simulink model "LKAS_AutoSave_20200909_1612"  (R2018b)
settings: Solver=FixedStepDiscrete  StartTime=0.0  StopTime=10.0  FixedStep=0.01  RelTol=1e-3
InitFcn:
  | tmpVer = ver('MATLAB');
  | tmpVer = str2num(tmpVer.Version);
  | % -------------------------------------------------------------------
  | %  MATLAB file generated by Simulink.saveVars on 21-Nov-2019 10:06:14
  | %  MATLAB version: 7.13.0.564 (R2011b)
  | % -------------------------------------------------------------------
  | 
  | 
  | SInt16 = Simulink.AliasType;
  | SInt16.Description = 'Num';
  | if (tmpVer > 7.11)
  | 	SInt16.DataScope = 'Auto';
  | end
  | SInt16.HeaderFile = 'Rte_Type.h';
  | SInt16.BaseType = 'int16';
  | 
  | SInt32 = Simulink.AliasType;
  | SInt32.Description = 'Num';
  | if (tmpVer > 7.11)
  | 	SInt32.DataScope = 'Auto';
  | end
  | SInt32.HeaderFile = 'Rte_Type.h';
  | SInt32.BaseType = 'int32';
  | 
  | SInt8 = Simulink.AliasType;
  | SInt8.Description = 'Num';
  | if (tmpVer > 7.11)
  | 	SInt8.DataScope = 'Auto';
  | end
  | SInt8.HeaderFile = 'Rte_Type.h';
  | SInt8.BaseType = 'int8';
  | 
  | T_A_m2_1024_1_u32 = Simulink.NumericType;
  | T_A_m2_1024_1_u32.Description = 'm2 (square meters  (m2))';
  | if (tmpVer > 7.11)
  | 	T_A_m2_1024_1_u32.DataScope = 'Auto';
  | end
  | T_A_m2_1024_1_u32.HeaderFile = 'Rte_Type.h';
  | T_A_m2_1024_1_u32.DataTypeMode = 'Fixed-point: slope and bias scaling';
  | T_A_m2_1024_1_u32.SignednessBool = false;
  | T_A_m2_1024_1_u32.WordLength = 32;
  | T_A_m2_1024_1_u32.FixedExponent = -10;
  | T_A_m2_1024_1_u32.SlopeAdjustmentFactor = 1;
  | T_A_m2_1024_1_u32.Bias = 0;
  | T_A_m2_1024_1_u32.DataTypeOverride = 'Inherit';
  | T_A_m2_1024_1_u32.IsAlias = true;
  | 
  | T_A_m2_65536_1_u16 = Simulink.NumericType;
  | T_A_m2_65536_1_u16.Description = 'm2 (square meters  (m2))';
  | if (tmpVer > 7.11)
  | 	T_A_m2_65536_1_u16.DataScope = 'Auto';
  | end
  | T_A_m2_65536_1_u16.HeaderFile = 'Rte_Type.h';
  | T_A_m2_65536_1_u16.DataTypeMode = 'Fixed-point: slope and bias scaling';
  | T_A_m2_65536_1_u16.SignednessBool = false;
  | T_A_m2_65536_1_u16.WordLength = 16;
  | T_A_m2_65536_1_u16.FixedExponent = -16;
  | T_A_m2_65536_1_u16.SlopeAdjustmentFactor = 1;
  | T_A_m2_65536_1_u16.Bias = 0;
  | T_A_m2_65536_1_u16.DataTypeOverride = 'Inherit';
  | ... (+4598 lines)
StopFcn:
  | clear  T_A_m2_1024_1_u32 T_A_m2_65536_1_u16 T_A_m2_Float32 T_A_mm2_10_1_u16 T_A_mm2_4_1_s16 T_A_mm2_Float32 T_Cnt_Num_10_1_u32 T_Cnt_Num_1_1_s16 T_Cnt_Num_1_1_s32 T_Cnt_Num_1_1_s8 T_Cnt_Num_1_1_u16 T_Cnt_Num_1_1_u32 T_Cnt_Num_1_1_u8 T_E_J_1_1_s32 T_E_J_Float32 T_E_kJ_128_1_s32 T_E_kJ_Float32 T_E_kwh_10_1_u16 T_E_kwh_Float32 T_Epl_kwhpkm_100_1_u16 T_Epl_kwhpkm_Float32 T_F_N_1_1_s16 T_F_N_Float32 T_I_A_1000_1_u16 T_I_A_1048576_1_s32 T_I_A_2048_1_s16 T_I_A_32_1_s16 T_I_A_Float32 T_I_mA_1_1_s16 T_I_mA_32768_128_s16 T_I_mA_Float32 T_J_kgpm2_128_1_u16 T_J_kgpm2_Float32 T_K_NA_1000_1_s16 T_K_NA_100_1_s16 T_K_NA_100_1_u16 T_K_NA_1024_1_s16 T_K_NA_1024_1_u16 T_K_NA_128_1_s16 T_K_NA_128_1_u16 T_K_NA_128_1_u8 T_K_NA_16777216_1_u32 T_K_NA_16_1_s16 T_K_NA_16_1_u16 T_K_NA_16_1_u8 T_K_NA_1_16_u16 T_K_NA_1_1_s16 T_K_NA_1_1_u16 T_K_NA_1_1_u8 T_K_NA_32768_1_s16 T_K_NA_32768_1_u16 T_K_NA_32_1_s8 T_K_NA_4096_1_u16 T_K_NA_4194304_1_s32 T_K_NA_4194304_1_u16 T_K_NA_65536_1_s32 T_K_NA_65536_1_u16 T_K_NA_8192_1_s16 T_K_NA_8_1_s16 T_K_NA_Float32 T_M_Nm_16_1_s16 T_M_Nm_1_1_s16 T_M_Nm_32768_1_s16 T_M_Nm_32_1_s16 T_M_Nm_4_1_s16 T_M_Nm_512_1_s16 T_M_Nm_Float32 T_P_W_1_4_s16 T_P_W_1_8_s16 T_P_W_Float32 T_P_kW_128_1_s16 T_P_kW_1_8_s16 T_P_kW_8_1_s32 T_P_kW_Float32 T_Pct_pct_1024_1_s32 T_Pct_pct_1024_1_u32 T_Pct_pct_10_1_s16 T_Pct_pct_10_1_u32 T_Pct_pct_128_100_s8 T_Pct_pct_1_1_s16 T_Pct_pct_1_4_u8 T_Pct_pct_255_100_u16 T_Pct_pct_255_100_u8 T_Pct_pct_256_1_s16 T_Pct_pct_256_1_u16 T_Pct_pct_65535_100_u16 T_Pct_pct_Float32 T_R_ohm_1024_1_s16 T_R_ohm_32_1_s16 T_R_ohm_Float32 T_TK_K_16_1_s16 T_TK_K_Float32 T_T_degC_10_400_1_u16 T_T_degC_16_1_s16 T_T_degC_1_40_1_u8 T_T_degC_2_80_1_u8 T_T_degC_Float32 T_U_V_1000_1_u16 T_U_V_10_1_u8 T_U_V_200_1_u8 T_U_V_32_1_s16 T_U_V_4096_1_s16 T_U_V_512_1_s16 T_U_V_65535_8_u16 T_U_V_8192_1_u16 T_U_V_Float32 T_U_mV_1_1_s16 T_U_mV_256_20_u16 T_U_mV_Float32 T_V_l_256_1_s16 T_V_l_4096_1_s16 T_V_l_64_1_s16 T_V_l_65535_100_u16 T_V_l_Float32 T_V_ml_128_1_s16 T_V_ml_1_1_s16 T_V_ml_32768_1_s16 T_V_ml_Float32 T_V_ul_32_1_u16 T_V_ul_Float32 T_Vpl_clpkm_512_1_u16 T_Vpl_clpkm_Float32 T_a_kphps_16_1_s16 T_a_kphps_Float32 T_a_mps2_128_1_s16 T_a_mps2_Float32 T_c_MJpkg_256_1_s16 T_c_MJpkg_Float32 T_c_kJpgpK_1024_1_s16 T_c_kJpgpK_Float32 T_c_kJpkgpK_128_1_u16 T_c_kJpkgpK_Float32 T_chrg_Ah_1_1_s16 T_chrg_Ah_1_1_u16 T_chrg_Ah_1_1_u8 T_chrg_Ah_256_1_u16 T_chrg_Ah_4194304_1_s32 T_chrg_Ah_512_1_u16 T_chrg_Ah_8_1_u16 T_chrg_Ah_Float32 T_cmp_NA_100_1_s16 T_cmp_NA_128_1_s16 T_cmp_NA_16_1_s16 T_cmp_NA_32768_1_u16 T_cmp_NA_Float32 T_d2n_rpmps2_4_1_s16 T_d2n_rpmps2_Float32 T_dPct_pctps_16_1_s16 T_dPct_pctps_256_1_s16 T_dPct_pctps_Float32 T_dT_degCps_128_1_s16 T_dT_degCps_Float32 T_dV_lph_1_1_s16 T_dV_lph_Float32 T_dV_lpm_128_1_s16 T_dV_lpm_32_1_s16 T_dV_lpm_Float32 T_dV_lps_1024_1_u16 T_dV_lps_4_1_u16 T_dV_lps_Float32 T_dV_mlps_1024_1_s16 T_dV_mlps_Float32 T_d_BitField16 T_dm_gps_128_1_s16 T_dm_gps_128_1_u16 T_dm_gps_256_1_u16 T_dm_gps_Float32 T_dm_mgps_1_1_s16 T_dm_mgps_Float32 T_dn_rpmps_1_1_s16 T_dn_rpmps_2_1_s16 T_dn_rpmps_Float32 T_dp_Paps_1_1_s16 T_dp_Paps_Float32 T_dp_kPaps_1_1_s16 T_dp_kPaps_8_1_s16 T_dp_kPaps_Float32 T_dphi_degps_128_1_s16 T_dphi_degps_8_1_s16 T_dphi_degps_Float32 T_dr_ps_256_1_s16 T_dr_ps_Float32 T_drho_mgplps_1_2_s16 T_drho_mgplps_Float32 T_e_NA_1_1_u8 T_f_Hz_1_1_u16 T_f_Hz_1_1_u32 T_f_Hz_64_1_u16 T_f_Hz_8_1_s16 T_f_Hz_Float32 T_g_BitField32 T_l_km_16_1_s16 T_l_km_1_1_u16 T_l_km_1_1_u32 T_l_km_Float32 T_l_m_1024_1_s16 T_l_m_16_1_s16 T_l_m_1_1_u32 T_l_m_Float32 T_l_mm_16_1_s16 T_l_mm_1_1_u16 T_l_mm_4096_1_s16 T_l_mm_4_1_u8 T_l_mm_64_1_s16 T_l_mm_Float32 T_m_g_1_1_s16 T_m_g_2048_1_s16 T_m_g_32_1_u16 T_m_g_Float32 T_m_kg_1024_1_s16 T_m_kg_1_1_s16 T_m_kg_1_1_u32 T_m_kg_Float32 T_m_mg_128_1_s16 T_m_mg_32_1_s16 T_m_mg_Float32 T_n_rpm_1_1_s16 T_n_rpm_1_25_u8 T_n_rpm_256_50_u16 T_n_rpm_2_25_u8 T_n_rpm_4_1_u16 T_n_rpm_Float32 T_p_MPa_64_1_s16 T_p_MPa_Float32 T_p_Pa_1_1_s16 T_p_Pa_Float32 T_p_kPa_1_10_u16 T_p_kPa_1_1_s16 T_p_kPa_1_1_u8 T_p_kPa_256_1_u16 T_p_kPa_32_1_u16 T_p_kPa_64_1_s16 T_p_kPa_Float32 T_phi_deg_100_1_s16 T_phi_deg_1024_1_s16 T_phi_deg_128_1_s16 T_phi_deg_1_1_u8 T_phi_deg_256_1_s16 T_phi_deg_2_1_s8 T_phi_deg_32_1_s16 T_phi_deg_512_6_s32 T_phi_deg_Float32 T_phi_rad_2048_1_s16 T_phi_rad_Float32 T_r_NA_1024_1_s16 T_r_NA_1024_1_u16 T_r_NA_16384_1_s16 T_r_NA_16_1_s16 T_r_NA_256_1_s8 T_r_NA_256_1_u16 T_r_NA_32768_1_u16 T_r_NA_32_1_u16 T_r_NA_4096_1_s16 T_r_NA_65535_2_u16 T_r_NA_8192_1_u16 T_r_NA_Float32 T_rho_gpl_8192_1_s16 T_rho_gpl_Float32 T_rho_kgpm3_16_1_s16 T_rho_kgpm3_Float32 T_rho_mgpl_1_1_s16 T_rho_mgpl_64_1_s16 T_rho_mgpl_Float32 T_t_hour_1_1_s16 T_t_hour_Float32 T_t_m_1_1_u16 T_t_m_Float32 T_t_ms_1_1_s16 T_t_ms_1_1_u16 T_t_ms_1_1_u32 T_t_ms_4096_1_s16 T_t_ms_64_1_s16 T_t_ms_Float32 T_t_s_1000_1_s16 T_t_s_100_1_s16 T_t_s_10_1_s16 T_t_s_10_1_u16 T_t_s_1_1_s16 T_t_s_1_1_u16 T_t_s_1_1_u32 T_t_s_Float32 T_t_us_10_1_u32 T_t_us_1_1_s16 T_t_us_1_1_u32 T_t_us_1_4_u16 T_t_us_Float32 T_v_kph_1_1_u8 T_v_kph_64_1_s16 T_v_kph_64_1_u16 T_v_kph_Float32 T_v_mps_256_1_s16 T_v_mps_Float32 T_w_radps_32_1_s16 T_w_radps_Float32 T_y_BitField8 T_y_BitFieldDiagProgress T_y_BitFieldDiagStatus T_y_NA_1_1_u8 SInt16 SInt32 SInt8 T_BOOLEAN UInt16 UInt32 UInt8 s16 s32 s8 u16 u32 u8
model workspace (MAT data in the model file):
  MCOS : class17 (value not decoded)
  MCOS : class17 (value not decoded)
  MCOS : class17 (value not decoded)
  MCOS : class17 (value not decoded)
  MCOS : class17 (value not decoded)
  MCOS : class17 (value not decoded)
  MCOS : class17 (value not decoded)
  MCOS : class17 (value not decoded)
  MCOS : class17 (value not decoded)
  MCOS : class17 (value not decoded)
  MCOS : class17 (value not decoded)
  MCOS : class17 (value not decoded)
  MCOS : class17 (value not decoded)
  MCOS : class17 (value not decoded)
  MCOS : class17 (value not decoded)
  MCOS : class17 (value not decoded)
  MCOS : class17 (value not decoded)
  MCOS : class17 (value not decoded)
  MCOS : class17 (value not decoded)
  MCOS : class17 (value not decoded)
  MCOS : class17 (value not decoded)
  MCOS : class17 (value not decoded)
  MCOS : class17 (value not decoded)
  MCOS : class17 (value not decoded)
  MCOS : class17 (value not decoded)
  MCOS : class17 (value not decoded)
  MCOS : class17 (value not decoded)
  MCOS : class17 (value not decoded)
  MCOS : class17 (value not decoded)
  MCOS : class17 (value not decoded)
  MCOS : class17 (value not decoded)
  MCOS : class17 (value not decoded)
  MCOS : class17 (value not decoded)
  MCOS : class17 (value not decoded)
  MCOS : class17 (value not decoded)
  MCOS : class17 (value not decoded)
  MCOS : class17 (value not decoded)
  MCOS : class17 (value not decoded)
  MCOS : class17 (value not decoded)
  MCOS : class17 (value not decoded)
  MCOS : class17 (value not decoded)
  MCOS : class17 (value not decoded)
  MCOS : class17 (value not decoded)
  MCOS : class17 (value not decoded)
  MCOS : class17 (value not decoded)
  MCOS : class17 (value not decoded)
  MCOS : class17 (value not decoded)
  MCOS : class17 (value not decoded)
  MCOS : class17 (value not decoded)
  MCOS : class17 (value not decoded)
  MCOS : class17 (value not decoded)
  MCOS : class17 (value not decoded)
  MCOS : class17 (value not decoded)
  MCOS : class17 (value not decoded)
  MCOS : class17 (value not decoded)
  MCOS : class17 (value not decoded)
  MCOS : class17 (value not decoded)
  MCOS : class17 (value not decoded)
  MCOS : class17 (value not decoded)
  MCOS : class17 (value not decoded)
  MCOS : class17 (value not decoded)
  MCOS : class17 (value not decoded)
  MCOS : class17 (value not decoded)
  MCOS : class17 (value not decoded)
  MCOS : class17 (value not decoded)
  MCOS : class17 (value not decoded)
  MCOS : class17 (value not decoded)
  MCOS : class17 (value not decoded)
  MCOS : class17 (value not decoded)
  MCOS : class17 (value not decoded)
  MCOS : class17 (value not decoded)
  MCOS : class17 (value not decoded)
  MCOS : class17 (value not decoded)
  MCOS : class17 (value not decoded)
  MCOS : class17 (value not decoded)
  MCOS : class17 (value not decoded)
  MCOS : class17 (value not decoded)
  MCOS : class17 (value not decoded)
  MCOS : class17 (value not decoded)
  MCOS : class17 (value not decoded)
  MCOS : class17 (value not decoded)
  MCOS : class17 (value not decoded)
  MCOS : class17 (value not decoded)
  MCOS : class17 (value not decoded)
  MCOS : class17 (value not decoded)
  MCOS : class17 (value not decoded)
  MCOS : class17 (value not decoded)
  MCOS : class17 (value not decoded)
  MCOS : class17 (value not decoded)
undefined symbols (not defined in the file): LKA_CarWidth, LKA_SampleTime, LKA_StrRatio_C, LKA_Veh2CamL_C, LKA_Veh2CamW_C, LKA_WhlBaseL_C, LL_CompSWA_C, LL_CrvtPrvwT_C, LL_DesDvt_C, LL_DvtComp_C, LL_DvtPrvwT_C, LL_DvtSpdDet_vDvtSpdMin_C, LL_HdAgExT_C, LL_HdAgPrvwT_C, LL_LAccMax_C, LL_LAccRMax_C, LL_LDW_EarliestWarnLine_C, LL_LDW_LatestWarnLine_C, LL_LDWS_SUPPRESS_HEADING, LL_LFClb_TFC_DiffCtlBalance, LL_LFClb_TFC_DiffCtrlMaxSWA, LL_LFClb_TFC_DiffCtrlRatio, LL_LFClb_TFC_facmGainLutGain1_C, LL_LFClb_TFC_facmGainLutGain2_C, LL_LFClb_TFC_facmIntegRatio, LL_LFClb_TFC_facmKlat_C, LL_LFClb_TFC_FfCtlRatio_C, LL_LFClb_TFC_phiIntegCtlMaxSWA_C, LL_LFClb_TFC_tiKlatPrvwT_C, LL_LFClb_TFC_vGainLutVehSpdLwr_C, LL_LFClb_TFC_vGainLutVehSpdUpr_C, LL_LKA_EarliestWarnLine_C, LL_LKA_LatestWarnLine_C, LL_LKAExPrcs_ExitC0Dvt, LL_LKAExPrcs_ExitC0Swt, LL_LKAExPrcs_tiExitTime1, LL_LKAExPrcs_tiExitTime2, LL_LKAExPrcs_tiExitTime3, LL_LKAS_OUT_OF_CONTROL_LAT_VEL, LL_LKAS_OUT_OF_CONTROL_TTLC, LL_LKASWASyn_M0, LL_LKASWASyn_M1, LL_LKASWASyn_M2, LL_LKASWASyn_M3K, LL_LKASWASyn_SWAaddMax, LL_LKASWASyn_T2, LL_LKASWASyn_tiTrqSwaRtTime, LL_LKASWASyn_tiTrqSwaTime, LL_LKASWASyn_TrqMax, LL_LKASWASyn_TrqSwaAddSwt, LL_LKASWASyn_TrqSwaRateDiff, LL_LSpdCompT_C, LL_lStpLngth_C, LL_MAX_DELAY_EPSSTAR_TIME, LL_MAX_DRIVER_TORQUE_DISABLE, LL_MAX_DRIVER_TORQUE_ENABLE, LL_MAX_LANE_WIDTH_DISABLE, LL_MAX_LANE_WIDTH_ENABLE, LL_MAX_LAT_ACC_DISABLE, LL_MAX_LAT_ACC_ENABLE ... (+29)
libraries: simulink x134, dspstat3 x3, simulink_extras x1
(part 8 of 19)

== system LKAS_AutoSave_20200909_1612/LKAS/LL/LL Inputs Mapping/bsLaneInfo/LanesReconstruct /Left 1Lane Reconstruct (Lft1LaneR) ==
  stFlag : Inport
  bsL1Info : Inport  Port=2
  Bus Creator2 : BusCreator  Inputs=10
  Bus Selector1 : BusSelector  OutputSignals=L1_C0,L1_C1,L1_C2,L1_C3,L1_VR,L1_Q,L1_Type,L1_W,L1_TLC,L1_LC
  Constant : Constant  Value=0  OutDataTypeStr=uint16
  Switch3 : Switch  Criteria=u2 > Threshold
  bsL1InfoR : Outport
  wires:
  Bus Selector1/9 -> Bus Creator2/9  "<L1_TLC>"
  Bus Selector1/10 -> Bus Creator2/10  "<L1_LC>"
  Bus Selector1/8 -> Bus Creator2/8  "<L1_W>"
  Bus Selector1/7 -> Bus Creator2/7  "<L1_Type>"
  Bus Selector1/5 -> Bus Creator2/5  "<L1_VR>"
  bsL1Info/1 -> Bus Selector1/1
  stFlag/1 -> Switch3/2
  Bus Selector1/6 -> Switch3/1  "<L1_Q>"
  Constant/1 -> Switch3/3
  Switch3/1 -> Bus Creator2/6  "L1_Q"
  Bus Creator2/1 -> bsL1InfoR/1  "bsL1Info"
  Bus Selector1/4 -> Bus Creator2/4  "<L1_C3>"
  Bus Selector1/3 -> Bus Creator2/3  "<L1_C2>"
  Bus Selector1/2 -> Bus Creator2/2  "<L1_C1>"
  Bus Selector1/1 -> Bus Creator2/1  "<L1_C0>"

== system LKAS_AutoSave_20200909_1612/LKAS/LL/LL Inputs Mapping/bsLaneInfo/LanesReconstruct /Left Lane Reconstruct (LftLaneR) ==
  lRoadW : Inport
  bsR0Info : Inport  Port=2
  bsL0Info : Inport  Port=3
  Add : Sum  Inputs=+-  OutDataTypeStr=single
  Bus Creator : BusCreator  Inputs=10
  Bus Selector1 : BusSelector  OutputSignals=L0_Q
  Bus Selector3 : BusSelector  OutputSignals=R0_C0,R0_C1,R0_C2,R0_C3,R0_VR,R0_Type,R0_W,R0_TLC,R0_LC
  Cast To Single{1..4,6..7} (6 alike) : DataTypeConversion  OutDataTypeStr=single  LockScale=on
  Cast To Single5 : DataTypeConversion  OutDataTypeStr=uint8  LockScale=on
  Cast To Single8 : DataTypeConversion  OutDataTypeStr=uint8  LockScale=on
  Gain : Gain  Gain=-1  OutDataTypeStr=Inherit: Same as input
  bsL0InfoR : Outport
  wires:
  Cast To Single7/1 -> Bus Creator/9  "L0_TLC"
  Cast To Single8/1 -> Bus Creator/10  "L0_LC"
  Cast To Single4/1 -> Bus Creator/5  "L0_VR"
  Cast To Single6/1 -> Bus Creator/8  "L0_W"
  Cast To Single5/1 -> Bus Creator/7  "L0_Type"
  Bus Selector3/8 -> Cast To Single7/1  "<R0_TLC>"
  Bus Selector3/9 -> Cast To Single8/1  "<R0_LC>"
  Bus Selector3/7 -> Cast To Single6/1  "<R0_W>"
  Bus Selector3/6 -> Cast To Single5/1  "<R0_Type>"
  lRoadW/1 -> Add/1
  bsR0Info/1 -> Bus Selector3/1
  Bus Selector3/1 -> Add/2  "<R0_C0>"
  Add/1 -> Gain/1
  Bus Selector3/2 -> Cast To Single1/1  "<R0_C1>"
  Bus Selector3/3 -> Cast To Single2/1  "<R0_C2>"
  Bus Selector3/4 -> Cast To Single3/1  "<R0_C3>"
  Bus Selector3/5 -> Cast To Single4/1  "<R0_VR>"
  bsL0Info/1 -> Bus Selector1/1
  Bus Selector1/1 -> Bus Creator/6  "<L0_Q>"
  Gain/1 -> Bus Creator/1  "L0_C0"
  Cast To Single1/1 -> Bus Creator/2  "L0_C1"
  Cast To Single2/1 -> Bus Creator/3  "L0_C2"
  Cast To Single3/1 -> Bus Creator/4  "L0_C3"
  Bus Creator/1 -> bsL0InfoR/1  "bsL0Info"

== system LKAS_AutoSave_20200909_1612/LKAS/LL/LL Inputs Mapping/bsLaneInfo/LanesReconstruct /Right 1Lane Reconstruct (Rgt1LaneR) ==
  stFlag : Inport
  bsR1Info : Inport  Port=2
  Bus Creator3 : BusCreator  Inputs=10
  Bus Selector1 : BusSelector  OutputSignals=R1_C0,R1_C1,R1_C2,R1_C3,R1_VR,R1_Q,R1_Type,R1_W,R1_TLC,R1_LC
  Constant : Constant  Value=0  OutDataTypeStr=uint16
  Switch3 : Switch  Criteria=u2 > Threshold
  bsL1InfoR : Outport
  wires:
  Bus Selector1/9 -> Bus Creator3/9  "<R1_TLC>"
  Bus Selector1/10 -> Bus Creator3/10  "<R1_LC>"
  Bus Selector1/8 -> Bus Creator3/8  "<R1_W>"
  Bus Selector1/7 -> Bus Creator3/7  "<R1_Type>"
  Bus Selector1/5 -> Bus Creator3/5  "<R1_VR>"
  Bus Selector1/1 -> Bus Creator3/1  "<R1_C0>"
  Bus Selector1/2 -> Bus Creator3/2  "<R1_C1>"
  Bus Selector1/3 -> Bus Creator3/3  "<R1_C2>"
  Bus Selector1/4 -> Bus Creator3/4  "<R1_C3>"
  Constant/1 -> Switch3/3
  Bus Selector1/6 -> Switch3/1  "<R1_Q>"
  stFlag/1 -> Switch3/2
  bsR1Info/1 -> Bus Selector1/1
  Bus Creator3/1 -> bsL1InfoR/1  "bsR1Info"
  Switch3/1 -> Bus Creator3/6  "R1_Q"

== system LKAS_AutoSave_20200909_1612/LKAS/LL/LL Inputs Mapping/bsLaneInfo/LanesReconstruct /Right Lane Reconstruct (RgtLaneR) ==
  bsL0Info : Inport
  bsR0Info : Inport  Port=2
  lRoadW : Inport  Port=3
  Add : Sum  OutDataTypeStr=single
  Bus Creator1 : BusCreator  Inputs=10
  Bus Selector1 : BusSelector  OutputSignals=R0_Q
  Bus Selector3 : BusSelector  OutputSignals=L0_C0,L0_C1,L0_C2,L0_C3,L0_VR,L0_Type,L0_W,L0_TLC,L0_LC
  Cast To Single{1..4,6..7} (6 alike) : DataTypeConversion  OutDataTypeStr=single  LockScale=on
  Cast To Single5 : DataTypeConversion  OutDataTypeStr=uint8  LockScale=on
  Cast To Single8 : DataTypeConversion  OutDataTypeStr=uint8  LockScale=on
  bsR0InfoR : Outport
  wires:
  Cast To Single7/1 -> Bus Creator1/9  "R0_TLC"
  Cast To Single6/1 -> Bus Creator1/8  "R0_W"
  Cast To Single8/1 -> Bus Creator1/10  "R0_LC"
  Cast To Single5/1 -> Bus Creator1/7  "R0_Type"
  Bus Selector3/8 -> Cast To Single7/1  "<L0_TLC>"
  Bus Selector3/9 -> Cast To Single8/1  "<L0_LC>"
  Bus Selector3/7 -> Cast To Single6/1  "<L0_W>"
  Bus Selector3/6 -> Cast To Single5/1  "<L0_Type>"
  Bus Selector3/1 -> Add/2  "<L0_C0>"
  bsL0Info/1 -> Bus Selector3/1
  lRoadW/1 -> Add/1
  Bus Selector3/2 -> Cast To Single1/1  "<L0_C1>"
  Bus Selector3/3 -> Cast To Single2/1  "<L0_C2>"
  Bus Selector3/4 -> Cast To Single3/1  "<L0_C3>"
  Bus Selector3/5 -> Cast To Single4/1  "<L0_VR>"
  bsR0Info/1 -> Bus Selector1/1
  Bus Selector1/1 -> Bus Creator1/6  "<R0_Q>"
  Bus Creator1/1 -> bsR0InfoR/1  "bsR0Info"
  Add/1 -> Bus Creator1/1  "R0_C0"
  Cast To Single1/1 -> Bus Creator1/2  "R0_C1"
  Cast To Single2/1 -> Bus Creator1/3  "R0_C2"
  Cast To Single3/1 -> Bus Creator1/4  "R0_C3"
  Cast To Single4/1 -> Bus Creator1/5  "R0_VR"

== system LKAS_AutoSave_20200909_1612/LKAS/LL/LL Inputs Mapping/bsLaneInfo/LanesReconstruct /RoadSide Offset ==
  bsL0Info : Inport
  bsR0Info : Inport  Port=2
  Abs : Abs
  Add : Sum
  Add1 : Sum  Inputs=+-
  Add2 : Sum
  Average Filter (AvrgFlt) : Subsystem
      mask Display:
      | port_label('input', 1, 'In');
      | port_label('input', 2, 'PtsNum');
      | port_label('output', 1, 'Out');
      | color('blue');
      | text(0.98,0.9,'VCDC Block','horizontalAlignment','right');
      | color('black');
      | text(0.5,0.55,'Average Filter','horizontalAlignment','center');
      | text(0.5,0.4,'(AvrgFlt)','horizontalAlignment','center');
  Average Filter (AvrgFlt)1 : Subsystem
      mask Display:
      | port_label('input', 1, 'In');
      | port_label('input', 2, 'PtsNum');
      | port_label('output', 1, 'Out');
      | color('blue');
      | text(0.98,0.9,'VCDC Block','horizontalAlignment','right');
      | color('black');
      | text(0.5,0.55,'Average Filter','horizontalAlignment','center');
      | text(0.5,0.4,'(AvrgFlt)','horizontalAlignment','center');
  Bus Creator1 : BusCreator  Inputs=10
  Bus Creator2 : BusCreator  Inputs=10
  Bus Selector1 : BusSelector  OutputSignals=R0_C0,R0_C1,R0_C2,R0_C3,R0_VR,R0_Q,R0_Type,R0_W,R0_TLC,R0_LC
  Bus Selector3 : BusSelector  OutputSignals=L0_C0,L0_C1,L0_C2,L0_C3,L0_VR,L0_Q,L0_Type,L0_W,L0_TLC,L0_LC
  Compare To Constant : simulink/Logic and Bit Operations/Compare To Constant  relop===  const=2  OutDataTypeStr=boolean
  Compare To Constant1 : simulink/Logic and Bit Operations/Compare To Constant  relop===  const=2  OutDataTypeStr=boolean
  PtsNum : Constant  Value=10  OutDataTypeStr=single
  PtsNum1 : Constant  Value=10  OutDataTypeStr=single
  Road Width Calculation (RoadWCal) : Subsystem
  Saturation : Saturate  UpperLimit=0.004  LowerLimit=0
  Switch : Switch  Criteria=u2 > Threshold
  Switch1 : Switch  Criteria=u2 > Threshold
  get_roadside_offset : MATLAB Function  TreatAsAtomicUnit=on
  bsL0Infoout : Outport
  bsR0Infoout : Outport  Port=2
  lRoadW : Outport  Port=3
  wires:
  Bus Selector3/9 -> Bus Creator1/9  "<L0_TLC>"
  Bus Creator1/1 -> bsL0Infoout/1  "bsL0Info"
  bsL0Info/1 -> Road Width Calculation (RoadWCal)/1(RoadWCal_L0Info), Bus Selector3/1
  Bus Selector3/1 -> Switch/3, Add/1  "<L0_C0>"
  Bus Selector3/2 -> Bus Creator1/2  "<L0_C1>"
  Bus Selector3/3 -> Bus Creator1/3, Add2/1  "<L0_C2>"
  Bus Selector3/4 -> Bus Creator1/4  "<L0_C3>"
  Bus Selector3/6 -> Bus Creator1/6  "<L0_Q>"
  Bus Selector3/5 -> Bus Creator1/5  "<L0_VR>"
  Bus Selector3/7 -> Bus Creator1/7, Compare To Constant/1  "<L0_Type>"
  Bus Selector3/8 -> Bus Creator1/8  "<L0_W>"
  Bus Selector3/10 -> Bus Creator1/10  "<L0_LC>"
  Compare To Constant/1 -> Switch/2
  [offset] -> Add/2
  Add/1 -> Switch/1
  Average Filter (AvrgFlt)/1(Out) -> Bus Creator1/1  "L0_C0"
  Bus Selector1/9 -> Bus Creator2/9  "<R0_TLC>"
  Bus Selector1/3 -> Bus Creator2/3, Add2/2  "<R0_C2>"
  bsR0Info/1 -> Road Width Calculation (RoadWCal)/2(RoadWCal_R0Info), Bus Selector1/1
  Bus Selector1/5 -> Bus Creator2/5  "<R0_VR>"
  Bus Selector1/2 -> Bus Creator2/2  "<R0_C1>"
  Bus Creator2/1 -> bsR0Infoout/1  "bsR0Info"
  Bus Selector1/4 -> Bus Creator2/4  "<R0_C3>"
  Bus Selector1/6 -> Bus Creator2/6  "<R0_Q>"
  Bus Selector1/10 -> Bus Creator2/10  "<R0_LC>"
  Bus Selector1/7 -> Bus Creator2/7, Compare To Constant1/1  "<R0_Type>"
  Add1/1 -> Switch1/1
  Bus Selector1/8 -> Bus Creator2/8  "<R0_W>"
  Average Filter (AvrgFlt)1/1(Out) -> Bus Creator2/1  "R0_C0"
  Compare To Constant1/1 -> Switch1/2
  [offset] -> Add1/2
  Bus Selector1/1 -> Switch1/3, Add1/1  "<R0_C0>"
  Road Width Calculation (RoadWCal)/1(RoadWCal_lRoadW) -> lRoadW/1, get_roadside_offset/2(lanewidth)
  Add2/1 -> Abs/1
  Abs/1 -> Saturation/1
  Saturation/1 -> get_roadside_offset/1(cur)
  get_roadside_offset/1(offset) -> [offset]
  Switch/1 -> Average Filter (AvrgFlt)/1(In)
  PtsNum/1 -> Average Filter (AvrgFlt)/2(PtsNum)
  Switch1/1 -> Average Filter (AvrgFlt)1/1(In)
  PtsNum1/1 -> Average Filter (AvrgFlt)1/2(PtsNum)

== system LKAS_AutoSave_20200909_1612/LKAS/LL/LLOn/LDW/Heading Angle Detection (HdAgDet)/If Action Subsystem ==
  In1 : Inport
  Action Port : ActionPort  InitializeStates=reset  ActionType=then
  Gain : Gain  Gain=-1  OutDataTypeStr=single
  rad to deg : Gain  Gain=180/pi  OutDataTypeStr=single
  Out1 : Outport  InitialOutput=0
  wires:
  In1/1 -> Gain/1
  Gain/1 -> rad to deg/1
  rad to deg/1 -> Out1/1

== system LKAS_AutoSave_20200909_1612/LKAS/LL/LLOn/LDW/Heading Angle Detection (HdAgDet)/If Action Subsystem1 ==
  In1 : Inport
  Action Port : ActionPort  InitializeStates=reset  ActionType=elseif
  rad to deg : Gain  Gain=180/pi  OutDataTypeStr=single
  Out1 : Outport  InitialOutput=0
  wires:
  In1/1 -> rad to deg/1
  rad to deg/1 -> Out1/1

== system LKAS_AutoSave_20200909_1612/LKAS/LL/LLOn/LDW/Heading Angle Detection (HdAgDet)/If Action Subsystem2 ==
  Action Port : ActionPort  InitializeStates=reset  ActionType=else
  Constant : Constant  Value=0  OutDataTypeStr=single
  Out1 : Outport  InitialOutput=0
  wires:
  Constant/1 -> Out1/1

== system LKAS_AutoSave_20200909_1612/LKAS/LL/LLOn/LDW/Heading Angle Detection (HdAgDet)/Sum Condition ==
  In : Inport
  Sum : Inport  Port=2
  state = reset : EnablePort  StatesWhenEnabling=reset
  Add1 : Sum  OutDataTypeStr=single
  Data Type Conversion : DataTypeConversion  OutDataTypeStr=uint8
  Memory : Memory  InheritSampleTime=on
  Relational Operator : RelationalOperator  OutDataTypeStr=boolean  RndMeth=Nearest
  Saturation : Saturate  UpperLimit=600  LowerLimit=0
  Out : Outport  OutputWhenDisabled=reset  InitialOutput=0
  wires:
  Relational Operator/1 -> Data Type Conversion/1
  Memory/1 -> Add1/2
  Add1/1 -> Saturation/1
  In/1 -> Add1/1
  Sum/1 -> Relational Operator/2
  Data Type Conversion/1 -> Out/1
  Saturation/1 -> Memory/1, Relational Operator/1

== system LKAS_AutoSave_20200909_1612/LKAS/LL/LLOn/LKA/Driver Torque Addition (DTA)/Subsystem ==
  DTA_bsInInfoSyn : Inport
  DTA_bsLFClb : Inport  Port=2
  LKA_SampleTime : Inport  Port=3
  Enable : EnablePort
  Add : Sum
  Bus Selector2 : BusSelector  OutputSignals=bsVehMovInfo.ESC_VehSpd,bsEPSInfo.EPS_SW_Trq,bsLaneInfo.bsL0Info.L0_C0,bsLaneInfo.bsR0Info.R0_C0
  Bus Selector4 : BusSelector  OutputSignals=LL_LKASWAClb.LL_LKASWASyn_SWAaddMax,LL_LKASWAClb.LL_LKASWASyn_TrqMax,LL_LKASWAClb.LL_LKASWASyn_TrqSwaAddSwt,LL_LKASWAClb.LL_LKASWASyn_tiTrqSwaTime,LL_LKASWAClb.LL_LKASWASyn_tiTrqSwaRtTime,LL_LKASWAClb.LL_LKASWASyn_TrqSwaRateDiff
  Constant1 : Constant  Value=5  OutDataTypeStr=single
  Constant2 : Constant  Value=-5  OutDataTypeStr=single
  Divide1 : Product  Inputs=***
  Divide3 : Product  Inputs=**
  DriverSwaTrqAdd : MATLAB Function  TreatAsAtomicUnit=on
  LowPass : Subsystem
  LowPass1 : Subsystem
  Rate Limiter Dynamic : simulink/Discontinuities/Rate Limiter Dynamic
      settings: SourceProductName=Simulink
  Saturation : Saturate  UpperLimit=30  LowerLimit=-30
  Out1 : Outport  OutputWhenDisabled=reset  InitialOutput=0
  wires:
  Add/1 -> Rate Limiter Dynamic/2
  Bus Selector4/3 -> Divide3/1, Divide1/1  "<LL_LKASWASyn_TrqSwaAddSwt>"
  LowPass1/1(y) -> Saturation/1  "SWARateAdd"
  Divide3/1 -> Add/1  "TrqSWAAdd"
  Constant2/1 -> Rate Limiter Dynamic/3
  Bus Selector4/1 -> DriverSwaTrqAdd/5(swaaddmax)  "<LL_LKASWASyn_SWAaddMax>"
  Constant1/1 -> Rate Limiter Dynamic/1
  DriverSwaTrqAdd/1(Swaadd) -> LowPass/2(u)  "TrqSWAAddRaw"
  Rate Limiter Dynamic/1 -> Out1/1
  Saturation/1 -> Divide1/2
  DTA_bsInInfoSyn/1 -> Bus Selector2/1
  Bus Selector4/4 -> LowPass/1(T)  "<LL_LKASWASyn_tiTrqSwaTime>"
  LowPass/1(y) -> Divide3/2, LowPass1/2(u)  "TrqSWAAdd"
  Divide1/1 -> Add/2  "SWARateAdd"
  Bus Selector2/2 -> DriverSwaTrqAdd/2(trq)  "<EPS_SW_Trq>"
  Bus Selector2/4 -> DriverSwaTrqAdd/4(r0c0)  "<R0_C0>"
  Bus Selector4/6 -> Divide1/3  "<LL_LKASWASyn_TrqSwaRateDiff>"
  Bus Selector2/1 -> DriverSwaTrqAdd/1(spd)  "<ESC_VehSpd>"
  Bus Selector4/5 -> LowPass1/1(T)  "<LL_LKASWASyn_tiTrqSwaRtTime>"
  Bus Selector2/3 -> DriverSwaTrqAdd/3(l0c0)  "<L0_C0>"
  LKA_SampleTime/1 -> LowPass/3(dT), LowPass1/3(dT)
  Bus Selector4/2 -> DriverSwaTrqAdd/6(trqmax)  "<LL_LKASWASyn_TrqMax>"
  DTA_bsLFClb/1 -> Bus Selector4/1

== system LKAS_AutoSave_20200909_1612/LKAS/LL/LLOn/LKA/Driver Torque Addition (DTA)/Subsystem1 ==
  DTA_bsInInfoSyn : Inport
  DTA_bsLFClb : Inport  Port=2
  Add1 : Sum  Inputs=-+
  Bus Selector : BusSelector  OutputSignals=bsEPSInfo.EPS_SW_Trq
  Bus Selector1 : BusSelector  OutputSignals=LL_LKASWAClb.LL_LKASWASyn_M3K,LL_LKASWAClb.LL_LKASWASyn_M0,LL_LKASWAClb.LL_LKASWASyn_M1,LL_LKASWAClb.LL_LKASWASyn_M2,LL_LKASWAClb.LL_LKASWASyn_T2
  Divide : Product  Inputs=**
  MATLAB Function : MATLAB Function  TreatAsAtomicUnit=on
  Moving Standard Deviation2 : Subsystem  TreatAsAtomicUnit=on
      mask Display: disp(['Moving' char(10) 'Standard' char(10) 'Deviation']);
  Saturation1 : Saturate  UpperLimit=0.2  LowerLimit=0
  Saturation2 : Saturate  UpperLimit=1  LowerLimit=0
  TickTime (TTime) : Subsystem
      mask Display:
      | port_label('output', 1, 'TTime');
      | color('blue');
      | text(0.98,0.9,'VCDC Block','horizontalAlignment','right');
      | color('black');
      | text(0.5,0.55,'Tick Time','horizontalAlignment','center');
      | text(0.5,0.4,'(TTime)','horizontalAlignment','center');
  Out1 : Outport
  wires:
  Bus Selector1/2 -> MATLAB Function/1(M0)  "<LL_LKASWASyn_M0>"
  Bus Selector1/3 -> MATLAB Function/2(M1)  "<LL_LKASWASyn_M1>"
  [PT1] -> MATLAB Function/4(T1)
  [T] -> MATLAB Function/6(T)
  Saturation1/1 -> Add1/1  "M3"
  MATLAB Function/1(M) -> Add1/2
  Bus Selector1/5 -> MATLAB Function/5(T2)  "<LL_LKASWASyn_T2>"
  TickTime (TTime)/1(Out1) -> [T]
  Divide/1 -> Saturation1/1
  Add1/1 -> Saturation2/1
  Bus Selector1/1 -> Divide/2  "<LL_LKASWASyn_M3K>"
  Bus Selector1/4 -> MATLAB Function/3(M2)  "<LL_LKASWASyn_M2>"
  Bus Selector/1 -> Moving Standard Deviation2/1(In1)  "<EPS_SW_Trq>"
  Moving Standard Deviation2/1(Out1) -> Divide/1
  DTA_bsInInfoSyn/1 -> Bus Selector/1
  DTA_bsLFClb/1 -> Bus Selector1/1
  Saturation2/1 -> Out1/1

== system LKAS_AutoSave_20200909_1612/LKAS/LL/LLOn/LKA/LKA Exit Processing (LKAExPrcs)/Exit Time 1 ==
  bsLKAInPInfo : Inport
  bsLKAClb : Inport  Port=2
  Abs : Abs
  Add : Sum
  Add2 : Sum  OutDataTypeStr=single
  Bus Selector1 : BusSelector  OutputSignals=LL_LKAExPrcs.LL_LKAExPrcs_tiExitTime1
  Bus Selector2 : BusSelector  OutputSignals=Pr_bsPrInfo.bsPrCrvtInfo.crPrvwCrvt
  Constant : Constant  Value=0.004  OutDataTypeStr=single
  Constant1 : Constant  Value=0.5  OutDataTypeStr=single
  Divide : Product  Inputs=***/
  Memory : Memory  InheritSampleTime=on
  Relational Operator4 : RelationalOperator  OutDataTypeStr=boolean  RndMeth=Nearest
  Saturation : Saturate  UpperLimit=0.004  LowerLimit=0
  Saturation2 : Saturate  UpperLimit=10  LowerLimit=0
  Exit1 : Outport
  wires:
  [LKA_SampleTime] -> Add2/1
  Add2/1 -> Saturation2/1, Relational Operator4/1
  bsLKAClb/1 -> Bus Selector1/1
  Saturation2/1 -> Memory/1
  Memory/1 -> Add2/2
  Relational Operator4/1 -> Exit1/1
  bsLKAInPInfo/1 -> Bus Selector2/1
  Constant/1 -> Divide/4
  Constant1/1 -> Divide/2
  Bus Selector2/1 -> Abs/1  "<crPrvwCrvt>"
  Divide/1 -> Add/2
  Abs/1 -> Saturation/1
  Add/1 -> Relational Operator4/2
  Saturation/1 -> Divide/3
  Bus Selector1/1 -> Add/1, Divide/1  "<LL_LKAExPrcs_tiExitTime1>"

== system LKAS_AutoSave_20200909_1612/LKAS/LL/LLOn/LKA/LKA Exit Processing (LKAExPrcs)/Exit Time 2 ==
  bsInInfoSyn : Inport
  bsLKAClb : Inport  Port=2
  bsLKAInPInfo : Inport  Port=3
  T1 : Inport  Port=4
  Abs : Abs
  Abs2 : Abs
  Abs3 : Abs
  Add : Sum
  Add1 : Sum
  Add2 : Sum  OutDataTypeStr=single
  Bus Selector : BusSelector  OutputSignals=LKA_Veh2CamW_C
  Bus Selector1 : BusSelector  OutputSignals=Pr_bsPrInfo.bsPrCrvtInfo.crPrvwCrvt
  Bus Selector2 : BusSelector  OutputSignals=bsLaneInfo.bsL0Info.L0_C0,bsLaneInfo.bsR0Info.R0_C0
  Bus Selector3 : BusSelector  OutputSignals=LL_LKAExPrcs.LL_LKAExPrcs_tiExitTime2
  Constant : Constant  Value=0.004  OutDataTypeStr=single
  Constant1 : Constant  Value=0.5  OutDataTypeStr=single
  Constant3 : Constant  Value=0.3  OutDataTypeStr=single
  Divide : Product  Inputs=***/
  Logical Operator1 : Logic  Inputs=3  AllPortsSameDT=off  OutDataTypeStr=boolean
  Memory : Memory  InheritSampleTime=on
  Relational Operator2 : RelationalOperator  OutDataTypeStr=boolean  RndMeth=Nearest
  Relational Operator3 : RelationalOperator  OutDataTypeStr=boolean  RndMeth=Nearest
  Relational Operator4 : RelationalOperator  OutDataTypeStr=boolean  RndMeth=Nearest
  Saturation : Saturate  UpperLimit=0.004  LowerLimit=0
  Saturation2 : Saturate  UpperLimit=10  LowerLimit=0
  Sum Condition1 : Subsystem
  Exit2 : Outport
  wires:
  Add/1 -> Relational Operator3/2, Relational Operator2/2
  Bus Selector2/2 -> Abs3/1  "<R0_C0>"
  Abs3/1 -> Relational Operator3/1
  Relational Operator2/1 -> Logical Operator1/2
  Bus Selector2/1 -> Abs2/1  "<L0_C0>"
  Abs2/1 -> Relational Operator2/1
  Relational Operator3/1 -> Logical Operator1/3
  Logical Operator1/1 -> Sum Condition1/Enable
  Constant3/1 -> Add/1
  Saturation2/1 -> Memory/1
  Relational Operator4/1 -> Logical Operator1/1
  Add2/1 -> Saturation2/1, Relational Operator4/1
  Memory/1 -> Add2/2
  [LKA_SampleTime] -> Add2/1
  T1/1 -> Relational Operator4/2
  Sum Condition1/1(Out) -> Exit2/1
  [LKA_SampleTime] -> Sum Condition1/1(Sample Time)
  bsInInfoSyn/1 -> Bus Selector2/1
  bsLKAInPInfo/1 -> Bus Selector1/1
  Bus Selector1/1 -> Abs/1  "<crPrvwCrvt>"
  Add1/1 -> Sum Condition1/2(Time Exit 2)
  Constant/1 -> Divide/4
  Abs/1 -> Saturation/1
  Constant1/1 -> Divide/2
  Divide/1 -> Add1/2
  Bus Selector3/1 -> Divide/1, Add1/1  "<LL_LKAExPrcs_tiExitTime2>"
  Saturation/1 -> Divide/3
  Bus Selector/1 -> Add/2  "<LKA_Veh2CamW_C>"
  [LKA_ConstantClb] -> Bus Selector/1
  bsLKAClb/1 -> Bus Selector3/1

== system LKAS_AutoSave_20200909_1612/LKAS/LL/LLOn/LKA/LKA Exit Processing (LKAExPrcs)/Exit Time 3 ==
  bsInInfoSyn : Inport
  bsLKAInPInfo : Inport  Port=2
  bsLKAClb : Inport  Port=3
  T1 : Inport  Port=4
  Abs2 : Abs
  Abs3 : Abs
  Abs4 : Abs
  Add : Sum
  Add2 : Sum  OutDataTypeStr=single
  Add4 : Sum
  Add5 : Sum  Inputs=+-
  Add6 : Sum
  Bus Selector : BusSelector  OutputSignals=LKA_Veh2CamW_C
  Bus Selector1 : BusSelector  OutputSignals=bsLaneInfo.bsL0Info.L0_C0,bsLaneInfo.bsR0Info.R0_C0
  Bus Selector2 : BusSelector  OutputSignals=bsLaneInfo.bsL0Info.L0_C0,bsLaneInfo.bsR0Info.R0_C0
  Bus Selector3 : BusSelector  OutputSignals=LL_LKAExPrcs.LL_LKAExPrcs_tiExitTime3,LL_LKAExPrcs.LL_LKAExPrcs_ExitC0Dvt,LL_LKAExPrcs.LL_LKAExPrcs_ExitC0Swt
  Bus Selector4 : BusSelector  OutputSignals=Pr_bsPrInfo.bsPrCrvtInfo.crPrvwCrvt
  Constant : Constant  Value=0.004  OutDataTypeStr=single
  Constant4 : Constant  Value=0.3  OutDataTypeStr=single
  Constant7 : Constant  Value=2  OutDataTypeStr=single
  Divide1 : Product  Inputs=**/
  Divide2 : Product  Inputs=*/
  Gain : Gain  Gain=0.25
  Logical Operator1 : Logic  Inputs=3  AllPortsSameDT=off  OutDataTypeStr=boolean
  Logical Operator2 : Logic  Inputs=4  AllPortsSameDT=off  OutDataTypeStr=boolean
  Memory : Memory  InheritSampleTime=on
  Moving Standard Deviation1 : Subsystem  TreatAsAtomicUnit=on
      mask Display: disp(['Moving' char(10) 'Standard' char(10) 'Deviation']);
  Moving Standard Deviation2 : Subsystem  TreatAsAtomicUnit=on
      mask Display: disp(['Moving' char(10) 'Standard' char(10) 'Deviation']);
  Relational Operator2 : RelationalOperator  OutDataTypeStr=boolean  RndMeth=Nearest
  Relational Operator3 : RelationalOperator  OutDataTypeStr=boolean  RndMeth=Nearest
  Relational Operator4 : RelationalOperator  OutDataTypeStr=boolean  RndMeth=Nearest
  Relational Operator5 : RelationalOperator  Operator=<=  OutDataTypeStr=boolean  RndMeth=Nearest
  Relational Operator6 : RelationalOperator  Operator=<=  OutDataTypeStr=boolean  RndMeth=Nearest
  Saturation : Saturate  UpperLimit=0.004  LowerLimit=0
  Saturation1 : Saturate  UpperLimit=5.5  LowerLimit=2.4
  Saturation2 : Saturate  UpperLimit=10  LowerLimit=0
  Sum Condition : Subsystem
  Sum Condition1 : Subsystem
  Exit3 : Outport
  wires:
  T1/1 -> Relational Operator4/2
  [LKA_SampleTime] -> Add2/1
  Memory/1 -> Add2/2
  Add2/1 -> Relational Operator4/1, Saturation2/1
  Relational Operator4/1 -> Logical Operator1/1
  Saturation2/1 -> Memory/1
  Add5/1 -> Add/1
  Logical Operator1/1 -> Logical Operator2/1
  Relational Operator3/1 -> Logical Operator1/3
  Abs2/1 -> Relational Operator2/1, Add4/1
  Bus Selector2/1 -> Abs2/1  "<L0_C0>"
  Relational Operator2/1 -> Logical Operator1/2
  Abs3/1 -> Add4/2, Relational Operator3/1
  Bus Selector2/2 -> Abs3/1  "<R0_C0>"
  Add/1 -> Relational Operator2/2, Relational Operator3/2
  Bus Selector3/1 -> Add6/1  "<LL_LKAExPrcs_tiExitTime3>"
  Bus Selector3/3 -> Logical Operator2/4  "<LL_LKAExPrcs_ExitC0Swt>"
  bsInInfoSyn/1 -> Bus Selector2/1, Bus Selector1/1
  Bus Selector3/2 -> Relational Operator5/2, Relational Operator6/2  "<LL_LKAExPrcs_ExitC0Dvt>"
  bsLKAClb/1 -> Bus Selector3/1
  Bus Selector1/2 -> Moving Standard Deviation1/1(In1)  "<R0_C0>"
  Bus Selector1/1 -> Moving Standard Deviation2/1(In1)  "<L0_C0>"
  Logical Operator2/1 -> Exit3/1
  Bus Selector/1 -> Add/2  "<LKA_Veh2CamW_C>"
  [LKA_ConstantClb] -> Bus Selector/1
  Moving Standard Deviation2/1(Out1) -> Relational Operator5/1
  Add4/1 -> Saturation1/1
  Saturation1/1 -> Gain/1
  Constant4/1 -> Add5/2
  Gain/1 -> Add5/1
  Relational Operator5/1 -> Sum Condition/Enable, Sum Condition/1(In)
  Sum Condition/1(Out) -> Logical Operator2/3
  Sum Condition1/1(Out) -> Logical Operator2/2
  Relational Operator6/1 -> Sum Condition1/Enable, Sum Condition1/1(In)
  Divide2/1 -> Sum Condition/2(In1), Sum Condition1/2(In1)
  Moving Standard Deviation1/1(Out1) -> Relational Operator6/1
  bsLKAInPInfo/1 -> Bus Selector4/1
  Constant/1 -> Divide1/3
  Divide1/1 -> Add6/2
  Abs4/1 -> Saturation/1
  Saturation/1 -> Divide1/2
  Bus Selector4/1 -> Abs4/1  "<crPrvwCrvt>"
  Constant7/1 -> Divide1/1
  [LKA_SampleTime] -> Divide2/2
  Add6/1 -> Divide2/1

== system LKAS_AutoSave_20200909_1612/LKAS/LL/LLOn/LKA/LKA Motion Planning (LKAMP) /LKA Motion Planning Calculation (LKAMPCal) ==
  LKAMPCal_bsLKAInPInfo : Inport
  LKAMPCal_bsLKAClb : Inport  Port=2
  LLClb_bsConstantClb : Inport  Port=3
  Action Port : ActionPort  InitializeStates=reset  ActionType=then
  Bus Creator : BusCreator  Inputs=6
  Bus Creator3 : BusCreator  Inputs=5
  Bus Creator5 : BusCreator  Inputs=3
  Bus Selector : BusSelector  OutputSignals=MPInP_stLDDir,MPInP_tiTTLCIni,MPInP_vVehSpdIni,MPInP_phiSWAIni,MPInP_phiPrvwHdAgIni,MPInP_phiHdAgIni,MPInP_phiHdAgMax,MPInP_lDvtIni,UndrLim_dphiSWARMax,StbFacm_SY
  Bus Selector1 : BusSelector  OutputSignals=LL_DesDvt_C,LL_lStpLngth_C
  Bus Selector2 : BusSelector  OutputSignals=LKA_WhlBaseL_C,LKA_StrRatio_C
  Bus Selector3 : BusSelector  OutputSignals=signal1,signal2,signal3,signal4,signal5
  Bus Selector4 : BusSelector  OutputSignals=LKA_WhlBaseL_C,LKA_StrRatio_C,StbFacm_SY
  MATLAB Function : MATLAB Function  TreatAsAtomicUnit=on
  Memory{,1..4} (5 alike) : Memory  InheritSampleTime=on
  Time Division (TDiv) : Subsystem
  Time Division (TDiv)1 : Subsystem
  Time Division (TDiv)2 : Subsystem
  Time Division (TDiv)3 : Subsystem
  Time Division (TDiv)4 : Subsystem
  LKAMPCal_bsLKAMPCalOut : Outport
  wires:
  Time Division (TDiv)4/1(Out2) -> Bus Creator3/5
  Time Division (TDiv)3/1(Out2) -> Bus Creator3/4
  Time Division (TDiv)2/1(Out2) -> Bus Creator3/3
  Time Division (TDiv)1/1(Out2) -> Bus Creator3/2
  Time Division (TDiv)/1(Out1) -> Bus Creator3/1
  Memory4/1 -> Time Division (TDiv)4/1(TDiv_bsTDivInfoOut1)
  MATLAB Function/11(K1K2Det_bsTDivInfoOut_Ph2SWAIni) -> Memory4/1
  MATLAB Function/10(K1K2Det_bsTDivInfoOut_Ph2DvtEnd) -> Memory3/1
  Memory3/1 -> Time Division (TDiv)3/1(TDiv_bsTDivInfoOut1)
  Memory2/1 -> Time Division (TDiv)2/1(TDiv_bsTDivInfoOut1)
  MATLAB Function/9(K1K2Det_bsTDivInfoOut_Mode2Num) -> Memory2/1
  MATLAB Function/8(K1K2Det_bsTDivInfoOut_Mode1Num) -> Memory1/1
  Memory1/1 -> Time Division (TDiv)1/1(TDiv_bsTDivInfoOut1)
  Bus Creator3/1 -> Bus Selector3/1
  Memory/1 -> Time Division (TDiv)/1(TDiv_bsTDivInfoOut)
  MATLAB Function/7(K1K2Det_bsTDivInfoOut_ModeFlg) -> Memory/1
  Bus Creator5/1 -> Bus Selector4/1
  Bus Selector4/2 -> MATLAB Function/20(K1K2Det_bsSysCfg_SY_StRatio_SY)  "<LKA_StrRatio_C>"
  Bus Selector4/3 -> MATLAB Function/21(K1K2Det_bsSysCfg_SY_StbFacm_SY)  "<StbFacm_SY>"
  Bus Selector4/1 -> MATLAB Function/19(K1K2Det_bsSysCfg_SY_WhlBase_SY)  "<LKA_WhlBaseL_C>"
  Bus Selector3/5 -> MATLAB Function/16(K1K2Det_bsTDivInfo_Ph2SWAIni)  "<signal5>"
  Bus Selector3/2 -> MATLAB Function/13(K1K2Det_bsTDivInfo_Mode1Num)  "<signal2>"
  Bus Selector3/1 -> MATLAB Function/12(K1K2Det_bsTDivInfo_ModeFlg)  "<signal1>"
  Bus Selector3/3 -> MATLAB Function/14(K1K2Det_bsTDivInfo_Mode2Num)  "<signal3>"
  Bus Selector3/4 -> MATLAB Function/15(K1K2Det_bsTDivInfo_Ph2DvtEnd)  "<signal4>"
  LLClb_bsConstantClb/1 -> Bus Selector2/1
  Bus Selector/9 -> MATLAB Function/10(K1K2Det_dphiSWARMax)  "<UndrLim_dphiSWARMax>"
  MATLAB Function/6(K1K2Det_dphi1PhHdAgIni) -> Bus Creator/6
  Bus Selector/5 -> MATLAB Function/5(K1K2Det_phiPrvwHdAgIni)  "<MPInP_phiPrvwHdAgIni>"
  Bus Selector/6 -> MATLAB Function/7(K1K2Det_phi1PhDesHdAgIni)  "<MPInP_phiHdAgIni>"
  Bus Selector/2 -> MATLAB Function/2(K1K2Det_tiTTLC0)  "<MPInP_tiTTLCIni>"
  MATLAB Function/4(K1K2Det_phi2PhSWAIni) -> Bus Creator/4  "K1K2Det_phi2PhSWAIni"
  Bus Selector/4 -> MATLAB Function/4(K1K2Det_phiIniSWA)  "<MPInP_phiSWAIni>"
  Bus Selector1/2 -> MATLAB Function/18(K1K2Det_lStpLngth)  "<LL_lStpLngth_C>"
  Bus Selector/8 -> MATLAB Function/9(K1K2Det_l1PhDvtIni)  "<MPInP_lDvtIni>"
  Bus Selector1/1 -> MATLAB Function/17(K1K2Det_lDesDvt)  "<LL_DesDvt_C>"
  Bus Selector/10 -> Bus Creator5/3  "<StbFacm_SY>"
  Bus Selector2/2 -> Bus Creator5/2  "<LKA_StrRatio_C>"
  Bus Selector2/1 -> Bus Creator5/1  "<LKA_WhlBaseL_C>"
  Bus Selector/1 -> MATLAB Function/1(K1K2Det_stLDDir)  "<MPInP_stLDDir>"
  Bus Selector/7 -> MATLAB Function/8(K1K2Det_phi2PhDesHdAg)  "<MPInP_phiHdAgMax>"
  Bus Selector/3 -> MATLAB Function/3(K1K2Det_vVehSpd)  "<MPInP_vVehSpdIni>"
  MATLAB Function/1(K1K2Det_dphi1PhSWAGrad) -> Bus Creator/1
  MATLAB Function/3(K1K2Det_dphi2PhSWAGrad2) -> Bus Creator/3
  MATLAB Function/5(K1K2Det_stReplFlag) -> Bus Creator/5
  MATLAB Function/2(K1K2Det_dphi2PhSWAGrad1) -> Bus Creator/2
  Bus Creator/1 -> LKAMPCal_bsLKAMPCalOut/1  "LKAMPCal_bsLKAMPCalOut"
  LKAMPCal_bsLKAClb/1 -> Bus Selector1/1
  LKAMPCal_bsLKAInPInfo/1 -> Bus Selector/1

== system LKAS_AutoSave_20200909_1612/LKAS/LL/LLOn/LKA/LKA Motion Planning (LKAMP) /Motion Planning Input Processing (MPInP) ==
  MPInP_stLKAActvFlg : Inport
  MPInP_phiHdAgMax : Inport  Port=2
  MPInP_bsLKAInPInfo : Inport  Port=3
  MPInP_bsInInfoSyn : Inport  Port=4
  Bus Creator : BusCreator  Inputs=11
  Bus Selector1 : BusSelector  OutputSignals=TTLC_bsTTLCInfo.LFTTTLC,TTLC_bsTTLCInfo.RGTTTLC
  Bus Selector3 : BusSelector  OutputSignals=bsSWAInfo.SW_Angle,bsVehMovInfo.ESC_VehSpd
  Bus Selector4 : BusSelector  OutputSignals=Pr_bsPrInfo.bsPrHdAgInfo.phiPrvwTTLCHdAg,Pr_bsPrInfo.bsPrDvtInfo.lDvt,Pr_bsPrInfo.bsPrHdAgInfo.phiHdAg,UndrLim_dphiSWARMax
  Cast To Single1 : DataTypeConversion  LockScale=on
  Lane Information Selection (LaneInfoSel) : Subsystem
  Lookup Table2 : Lookup_n-D  NumberOfTableDimensions=1  BreakpointsForDimension1=[11.7,18.83,26.98,31.98,51.04,79,86.08,90.59]  BeginIndexSearchUsingPreviousIndexResult=on  Table=[0.012141,0.005179,0.00298,0.002547,0.001715,0.001283,0.001021,0.000982]  RemoveProtectionInput=on  InternalRulePriority=Speed  OutDataTypeStr=single  InputSameDT=on
  MATLAB Function : MATLAB Function  TreatAsAtomicUnit=on
  Saturation : Saturate  UpperLimit=20  LowerLimit=-20
  Saturation1 : Saturate  UpperLimit=0.0117  LowerLimit=0.00237
  Saturation2 : Saturate  UpperLimit=2  LowerLimit=0.6
  Signal Latching2 : Subsystem  mask(Signal Latching:){LatchTime=1}
      mask prompts: LatchTime "Latch time(-):"
      mask help:
      | If the latch time is not reached, the input signal will just go through the block. If the latch time is reached, the output will be held and do not change again. The latch time is described with the number of the sampling time.
      | ----vcdc.ascl@jlu 19-01-15
  Signal Latching3 : Subsystem  mask(Signal Latching:){LatchTime=1}
      mask prompts: LatchTime "Latch time(-):"
      mask help:
      | If the latch time is not reached, the input signal will just go through the block. If the latch time is reached, the output will be held and do not change again. The latch time is described with the number of the sampling time.
      | ----vcdc.ascl@jlu 19-01-15
  Signal Latching4 : Subsystem  mask(Signal Latching:){LatchTime=1}
      mask prompts: LatchTime "Latch time(-):"
      mask help:
      | If the latch time is not reached, the input signal will just go through the block. If the latch time is reached, the output will be held and do not change again. The latch time is described with the number of the sampling time.
      | ----vcdc.ascl@jlu 19-01-15
  Signal Latching5 : Subsystem  mask(Signal Latching:){LatchTime=1}
      mask prompts: LatchTime "Latch time(-):"
      mask help:
      | If the latch time is not reached, the input signal will just go through the block. If the latch time is reached, the output will be held and do not change again. The latch time is described with the number of the sampling time.
      | ----vcdc.ascl@jlu 19-01-15
  Signal Latching6 : Subsystem  mask(Signal Latching:){LatchTime=1}
      mask prompts: LatchTime "Latch time(-):"
      mask help:
      | If the latch time is not reached, the input signal will just go through the block. If the latch time is reached, the output will be held and do not change again. The latch time is described with the number of the sampling time.
      | ----vcdc.ascl@jlu 19-01-15
  Signal Latching7 : Subsystem  mask(Signal Latching:){LatchTime=1}
      mask prompts: LatchTime "Latch time(-):"
      mask help:
      | If the latch time is not reached, the input signal will just go through the block. If the latch time is reached, the output will be held and do not change again. The latch time is described with the number of the sampling time.
      | ----vcdc.ascl@jlu 19-01-15
  Subsystem : Subsystem
  MPInP_bsMPInPInfo : Outport
  wires:
  Saturation/1 -> MATLAB Function/3(phiFf)
  [Ff] -> Saturation/1
  [ActFlg] -> MATLAB Function/1(Actflg)
  Signal Latching6/1(Out) -> Bus Creator/8  "MPInP_phiSWAIni"
  Bus Selector4/1 -> Signal Latching2/1(In)  "<phiPrvwTTLCHdAg>"
  Bus Selector4/4 -> Bus Creator/6  "<UndrLim_dphiSWARMax>"
  Bus Selector1/2 -> Lane Information Selection (LaneInfoSel)/3(LaneInfoSel_facmRgtLane)  "<RGTTTLC>"
  Bus Selector1/1 -> Lane Information Selection (LaneInfoSel)/2(LaneInfoSel_facmLftLane)  "<LFTTTLC>"
  Lane Information Selection (LaneInfoSel)/1(LaneInfoSel_facmActvLane) -> Signal Latching5/1(In)
  MPInP_bsLKAInPInfo/1 -> Bus Selector1/1, Bus Selector4/1
  Cast To Single1/1 -> Bus Creator/10  "MPInP_vVehSpd"
  Bus Selector4/3 -> Signal Latching4/1(In)  "<phiHdAg>"
  Bus Selector3/1 -> Signal Latching6/1(In), MATLAB Function/2(phiSWA)  "<SW_Angle>"
  MPInP_phiHdAgMax/1 -> Bus Creator/7  "MPInP_phiHdAgMax"
  Bus Selector4/2 -> Signal Latching3/1(In)  "<lDvt>"
  Signal Latching4/1(Out) -> Bus Creator/5  "MPInP_phiHdAgIni"
  Signal Latching2/1(Out) -> Bus Creator/3  "MPInP_phiPrvwHdAgIni"
  Signal Latching3/1(Out) -> Bus Creator/4  "MPInP_lDvtIni"
  MPInP_stLKAActvFlg/1 -> Subsystem/1(In1), Lane Information Selection (LaneInfoSel)/1(LaneInfoSel_stLKAActvFlg)
  Saturation1/1 -> Bus Creator/11  "StbFacm_SY"
  Signal Latching5/1(Out) -> Saturation2/1  "MPInP_tiTTLCIni"
  Signal Latching7/1(Out) -> Bus Creator/9  "MPInP_vVehSpdIni"
  Bus Selector3/2 -> Signal Latching7/1(In), Cast To Single1/1, Lookup Table2/1  "<ESC_VehSpd>"
  MPInP_bsInInfoSyn/1 -> Bus Selector3/1
  Subsystem/1(Out6) -> Bus Creator/1  "MPInP_stLDDir"
  Lookup Table2/1 -> Saturation1/1
  Bus Creator/1 -> MPInP_bsMPInPInfo/1
  Saturation2/1 -> Bus Creator/2  "MPInP_tiTTLCIni"

== system LKAS_AutoSave_20200909_1612/LKAS/LL/LLOn/LKA/LKA Motion Planning (LKAMP) /Nominal Time Calculation (NomTCalc) ==
  NomTCalc_vVehSpd : Inport
  NomTCalc_vVehSpdIni : Inport  Port=2
  Add : Sum  OutDataTypeStr=single
  Divide : Product  Inputs=*/  OutDataTypeStr=single
  Gain : Gain  Gain=1/3.6  OutDataTypeStr=single
  Gain1 : Gain  Gain=1/3.6  OutDataTypeStr=single
  Memory : Memory  InheritSampleTime=on
  Product : Product
  NomTCalc_tiNomT : Outport
  wires:
  [LKA_SampleTime] -> Product/2
  Divide/1 -> Add/1
  Product/1 -> Divide/1
  Gain1/1 -> Divide/2
  NomTCalc_vVehSpdIni/1 -> Gain1/1
  Gain/1 -> Product/1
  Memory/1 -> Add/2
  Add/1 -> Memory/1, NomTCalc_tiNomT/1
  NomTCalc_vVehSpd/1 -> Gain/1

== system LKAS_AutoSave_20200909_1612/LKAS/LL/LLOn/LKA/LKA Motion Planning (LKAMP) /Steering Wheel Angle Command Calculation (SWACmdCal) ==
  SWACmdCal_bsK1K2DetOut : Inport
  SWACmdCal_bsLKAInPInfo : Inport  Port=2
  SWACmdCal_tiNomT : Inport  Port=3
  Bus Selector : BusSelector  OutputSignals=K1K2Det_dphi1PhSWAGrad,K1K2Det_phi2PhSWAIni,K1K2Det_dphi2PhSWAGrad1
  Bus Selector1 : BusSelector  OutputSignals=MPInP_phiSWAIni
  SWACmd : MATLAB Function  TreatAsAtomicUnit=on
  SWACmdCal_phiSWACmd : Outport
  SWACmdCal_tiT1 : Outport  Port=2
  SWACmdCal_tiT2 : Outport  Port=3
  wires:
  SWACmd/3(T2) -> SWACmdCal_tiT2/1
  SWACmd/1(SWACmd_phiSWACmd) -> SWACmdCal_phiSWACmd/1
  SWACmdCal_bsK1K2DetOut/1 -> Bus Selector/1
  Bus Selector/2 -> SWACmd/2(SWACmd_phi2PhSWAIni)  "<K1K2Det_phi2PhSWAIni>"
  Bus Selector/3 -> SWACmd/3(SWACmd_dphi2PhSWAGrad)  "<K1K2Det_dphi2PhSWAGrad1>"
  Bus Selector/1 -> SWACmd/1(SWACmd_dphi1PhSWAGrad)  "<K1K2Det_dphi1PhSWAGrad>"
  SWACmdCal_bsLKAInPInfo/1 -> Bus Selector1/1
  Bus Selector1/1 -> SWACmd/4(SWACmd_phi1PhSWAIni)  "<MPInP_phiSWAIni>"
  SWACmdCal_tiNomT/1 -> SWACmd/5(SWACmd_tiNomT)
  SWACmd/2(T1) -> SWACmdCal_tiT1/1
